simulink model "FullCarLateral"  (R2023b)
settings: Solver=FixedStepAuto  StartTime=0.0  StopTime=30  FixedStep=dt  MaxStep=0.001  RelTol=1e-3
model workspace (MAT data in the model file):
  AMU : Simulink.Signal (value not decoded)
  EPSILON : Simulink.Signal (value not decoded)
  FZO : Simulink.Signal (value not decoded)
  LCX : Simulink.Signal (value not decoded)
  LCY : Simulink.Signal (value not decoded)
  LCZ : Simulink.Signal (value not decoded)
  LEX : Simulink.Signal (value not decoded)
  LEY : Simulink.Signal (value not decoded)
  LFZO : Simulink.Signal (value not decoded)
  LHX : Simulink.Signal (value not decoded)
  LHY : Simulink.Signal (value not decoded)
  LKXKAPPA : Simulink.Signal (value not decoded)
  LKYALPHA : Simulink.Signal (value not decoded)
  LKYGAMMA : Simulink.Signal (value not decoded)
  LKZGAMMA : Simulink.Signal (value not decoded)
  LMR : Simulink.Signal (value not decoded)
  LMUV : Simulink.Signal (value not decoded)
  LMUX : Simulink.Signal (value not decoded)
  LMUXAST : Simulink.Signal (value not decoded)
  LMUXPRIME : Simulink.Signal (value not decoded)
  LMUY : Simulink.Signal (value not decoded)
  LMUYAST : Simulink.Signal (value not decoded)
  LMUYPRIME : Simulink.Signal (value not decoded)
  LMX : Simulink.Signal (value not decoded)
  LMY : Simulink.Signal (value not decoded)
  LS : Simulink.Signal (value not decoded)
  LT : Simulink.Signal (value not decoded)
  LVX : Simulink.Signal (value not decoded)
  LVY : Simulink.Signal (value not decoded)
  LVYKAPPA : Simulink.Signal (value not decoded)
  LXALPHA : Simulink.Signal (value not decoded)
  LYKAPPA : Simulink.Signal (value not decoded)
  PCX1 : Simulink.Signal (value not decoded)
  PCY1 : Simulink.Signal (value not decoded)
  PDX1 : Simulink.Signal (value not decoded)
  PDX2 : Simulink.Signal (value not decoded)
  PDX3 : Simulink.Signal (value not decoded)
  PDY1 : Simulink.Signal (value not decoded)
  PDY2 : Simulink.Signal (value not decoded)
  PDY3 : Simulink.Signal (value not decoded)
  PEX1 : Simulink.Signal (value not decoded)
  PEX2 : Simulink.Signal (value not decoded)
  PEX3 : Simulink.Signal (value not decoded)
  PEX4 : Simulink.Signal (value not decoded)
  PEY1 : Simulink.Signal (value not decoded)
  PEY2 : Simulink.Signal (value not decoded)
  PEY3 : Simulink.Signal (value not decoded)
  PEY4 : Simulink.Signal (value not decoded)
  PEY5 : Simulink.Signal (value not decoded)
  PHX1 : Simulink.Signal (value not decoded)
  PHX2 : Simulink.Signal (value not decoded)
  PHY1 : Simulink.Signal (value not decoded)
  PHY2 : Simulink.Signal (value not decoded)
  PKX1 : Simulink.Signal (value not decoded)
  PKX2 : Simulink.Signal (value not decoded)
  PKX3 : Simulink.Signal (value not decoded)
  PKY1 : Simulink.Signal (value not decoded)
  PKY2 : Simulink.Signal (value not decoded)
  PKY3 : Simulink.Signal (value not decoded)
  PKY4 : Simulink.Signal (value not decoded)
  PKY5 : Simulink.Signal (value not decoded)
  PKY6 : Simulink.Signal (value not decoded)
  PKY7 : Simulink.Signal (value not decoded)
  PVX1 : Simulink.Signal (value not decoded)
  PVX2 : Simulink.Signal (value not decoded)
  PVY1 : Simulink.Signal (value not decoded)
  PVY2 : Simulink.Signal (value not decoded)
  PVY3 : Simulink.Signal (value not decoded)
  PVY4 : Simulink.Signal (value not decoded)
  QBZ1 : Simulink.Signal (value not decoded)
  QBZ10 : Simulink.Signal (value not decoded)
  QBZ2 : Simulink.Signal (value not decoded)
  QBZ3 : Simulink.Signal (value not decoded)
  QBZ5 : Simulink.Signal (value not decoded)
  QBZ6 : Simulink.Signal (value not decoded)
  QBZ9 : Simulink.Signal (value not decoded)
  QCZ1 : Simulink.Signal (value not decoded)
  QDZ1 : Simulink.Signal (value not decoded)
  QDZ10 : Simulink.Signal (value not decoded)
  QDZ11 : Simulink.Signal (value not decoded)
  QDZ2 : Simulink.Signal (value not decoded)
  QDZ3 : Simulink.Signal (value not decoded)
  QDZ4 : Simulink.Signal (value not decoded)
  QDZ6 : Simulink.Signal (value not decoded)
  QDZ7 : Simulink.Signal (value not decoded)
  QDZ8 : Simulink.Signal (value not decoded)
  QDZ9 : Simulink.Signal (value not decoded)
  QEZ1 : Simulink.Signal (value not decoded)
  QEZ2 : Simulink.Signal (value not decoded)
  QEZ3 : Simulink.Signal (value not decoded)
  QEZ4 : Simulink.Signal (value not decoded)
  QEZ5 : Simulink.Signal (value not decoded)
  QHZ1 : Simulink.Signal (value not decoded)
  QHZ2 : Simulink.Signal (value not decoded)
  QHZ3 : Simulink.Signal (value not decoded)
  QHZ4 : Simulink.Signal (value not decoded)
  QSX1 : Simulink.Signal (value not decoded)
  QSX2 : Simulink.Signal (value not decoded)
  QSX3 : Simulink.Signal (value not decoded)
  QX1 : Simulink.Signal (value not decoded)
  QX2 : Simulink.Signal (value not decoded)
  QX3 : Simulink.Signal (value not decoded)
  QX4 : Simulink.Signal (value not decoded)
  QX5 : Simulink.Signal (value not decoded)
  QX6 : Simulink.Signal (value not decoded)
  RBX1 : Simulink.Signal (value not decoded)
  RBX2 : Simulink.Signal (value not decoded)
  RBX3 : Simulink.Signal (value not decoded)
  RBY1 : Simulink.Signal (value not decoded)
  RBY2 : Simulink.Signal (value not decoded)
  RBY3 : Simulink.Signal (value not decoded)
  RBY4 : Simulink.Signal (value not decoded)
  RCX1 : Simulink.Signal (value not decoded)
  RCY1 : Simulink.Signal (value not decoded)
  REX1 : Simulink.Signal (value not decoded)
  REX2 : Simulink.Signal (value not decoded)
  REY1 : Simulink.Signal (value not decoded)
  REY2 : Simulink.Signal (value not decoded)
  RHX1 : Simulink.Signal (value not decoded)
  RHY1 : Simulink.Signal (value not decoded)
  RHY2 : Simulink.Signal (value not decoded)
  RO : Simulink.Signal (value not decoded)
  RVY1 : Simulink.Signal (value not decoded)
  RVY2 : Simulink.Signal (value not decoded)
  RVY3 : Simulink.Signal (value not decoded)
  RVY4 : Simulink.Signal (value not decoded)
  RVY5 : Simulink.Signal (value not decoded)
  RVY6 : Simulink.Signal (value not decoded)
  SSZ1 : Simulink.Signal (value not decoded)
  SSZ2 : Simulink.Signal (value not decoded)
  SSZ3 : Simulink.Signal (value not decoded)
  SSZ4 : Simulink.Signal (value not decoded)
  VCX : Simulink.Signal (value not decoded)
  ZETA0 : Simulink.Signal (value not decoded)
  ZETA1 : Simulink.Signal (value not decoded)
  ZETA2 : Simulink.Signal (value not decoded)
  ZETA3 : Simulink.Signal (value not decoded)
  ZETA4 : Simulink.Signal (value not decoded)
  ZETA5 : Simulink.Signal (value not decoded)
  ZETA6 : Simulink.Signal (value not decoded)
  ZETA7 : Simulink.Signal (value not decoded)
  ZETA8 : Simulink.Signal (value not decoded)
values from neighbouring files (symbols this model uses):
  A = load('PSS LATERAL FORCE COEFFS.mat').A    [FullCarLateralParams.m]
  B = load('PSS ALIGNING TORQUE COEFFS.mat').B    [FullCarLateralParams.m]
  b = 0.085    [FullCarLateralParams.m]
  C = load('COMBINED OVERTURNING MOMENT COEFFS.mat').C    [FullCarLateralParams.m]
  c_roll = 0.1    [FullCarLateralParams.m]
  cD = 1.23    [FullCarLateralParams.m]
  cL = 3.71    [FullCarLateralParams.m]
  D = load('PLS LONGITUDINAL FORCE COEFFS.mat').D    [FullCarLateralParams.m]
  dt = 0.001    [FullCarLateralParams.m]
  E = load('COMBINED LONGITUDINAL FORCE COEFFS.mat').E    [FullCarLateralParams.m]
  e_FL = atan(tf/lf)    [FullCarLateralParams.m]
  e_FR = atan(lf/tf)    [FullCarLateralParams.m]
  e_RL = atan(lr/tr)    [FullCarLateralParams.m]
  e_RR = atan(tr/lr)    [FullCarLateralParams.m]
  F = load('COMBINED LATERAL FORCE COEFFS.mat').F    [FullCarLateralParams.m]
  frontalA = 1    [FullCarLateralParams.m]
  g = 9.81    [FullCarLateralParams.m]
  G = load('COMBINED ALIGNING TORQUE COEFFS.mat').G    [FullCarLateralParams.m]
  gearboxEff = 0.95    [FullCarLateralParams.m]
  GR = 11.86    [FullCarLateralParams.m]
  hCG = 0.2    [FullCarLateralParams.m]
  Ix_wheel = (0.07829 + Ix_motor*GR*GR) * Ix_wheel_factor    (= 0.1168307304)    [FullCarLateralParams.m]
  Iz_vehicle = 125    [FullCarLateralParams.m]
  lf = wb - lr    (= 0.755)    [FullCarLateralParams.m]
  lowpassT = 0.05    [FullCarLateralParams.m]
  lr = 0.78    [FullCarLateralParams.m]
  m = 250    [FullCarLateralParams.m]
  motorOmegaLimit = 2094    [FullCarLateralParams.m]
  R_FL = sqrt(tf^2 + lf^2)    [FullCarLateralParams.m]
  R_FR = R_FL    [FullCarLateralParams.m]
  R_RL = sqrt(tr^2 + lr^2)    [FullCarLateralParams.m]
  R_RR = R_RL    [FullCarLateralParams.m]
  R_wheel = 0.2    [FullCarLateralParams.m]
  rho = 1.293    [FullCarLateralParams.m]
  tireFactor_X_Accel = 0.6    [FullCarLateralParams.m]
  tireFactor_X_Brake = 0.6    [FullCarLateralParams.m]
  tireFactor_Y = 1    [FullCarLateralParams.m]
  TLLTD = 0.5    [FullCarLateralParams.m]
  tr = trackWidth / 2    (= 0.6)    [FullCarLateralParams.m]
  trackWidth = 1.2    [FullCarLateralParams.m]
  wb = 1.535    [FullCarLateralParams.m]
  wheelSideBrakeFactor = 1    [FullCarLateralParams.m]
undefined symbols (not defined in the file or in its folder): trackReference
libraries: simulink_extras x11, eeGeneralControl x3, slpidlib x2, simulink x2
(part 6 of 6)

== matlab function FullCarLateral/Car/Tire Model Pacejka 5.2/Pacejka 5.2 FL3 ==
  settings: updateMethod=DISCRETE  sampleTime=dt
  data: SL input; FX output; SA input; FZ input; IA input; FY output; FZO data_store_memory; RO data_store_memory; VCX data_store_memory; PCY1 data_store_memory; PDY1 data_store_memory; PDY2 data_store_memory; PDY3 data_store_memory; PEY1 data_store_memory; PEY2 data_store_memory; PEY3 data_store_memory; PEY4 data_store_memory; PEY5 data_store_memory; PKY1 data_store_memory; PKY2 data_store_memory; PKY3 data_store_memory; PKY4 data_store_memory; PKY5 data_store_memory; PKY6 data_store_memory; PKY7 data_store_memory; PHY1 data_store_memory; PHY2 data_store_memory; PVY1 data_store_memory; PVY2 data_store_memory; PVY3 data_store_memory; PVY4 data_store_memory; PCX1 data_store_memory; PDX1 data_store_memory; PDX2 data_store_memory; PDX3 data_store_memory; PEX1 data_store_memory; PEX2 data_store_memory; PEX3 data_store_memory; PEX4 data_store_memory; PKX1 data_store_memory; PKX2 data_store_memory; PKX3 data_store_memory; PHX1 data_store_memory; PHX2 data_store_memory; PVX1 data_store_memory; PVX2 data_store_memory; QBZ1 data_store_memory; QBZ2 data_store_memory; QBZ3 data_store_memory; QBZ5 data_store_memory; QBZ6 data_store_memory; QBZ9 data_store_memory; QBZ10 data_store_memory; QCZ1 data_store_memory; QDZ1 data_store_memory; QDZ2 data_store_memory; QDZ3 data_store_memory; QDZ4 data_store_memory; QDZ6 data_store_memory; QDZ7 data_store_memory; QDZ8 data_store_memory; QDZ9 data_store_memory; QDZ10 data_store_memory; QDZ11 data_store_memory; QEZ1 data_store_memory; QEZ2 data_store_memory; QEZ3 data_store_memory; QEZ4 data_store_memory; QEZ5 data_store_memory; QHZ1 data_store_memory; QHZ2 data_store_memory; QHZ3 data_store_memory; QHZ4 data_store_memory; QSX1 data_store_memory; QSX2 data_store_memory; QSX3 data_store_memory; QX1 data_store_memory; QX2 data_store_memory; QX3 data_store_memory; QX4 data_store_memory; QX5 data_store_memory; QX6 data_store_memory; RBX1 data_store_memory; RBX2 data_store_memory; RBX3 data_store_memory; RCX1 data_store_memory; REX1 data_store_memory; REX2 data_store_memory; RHX1 data_store_memory; RBY1 data_store_memory; RBY2 data_store_memory; RBY3 data_store_memory; RBY4 data_store_memory; RCY1 data_store_memory; REY1 data_store_memory; REY2 data_store_memory; RHY1 data_store_memory; RHY2 data_store_memory; RVY1 data_store_memory; RVY2 data_store_memory; RVY3 data_store_memory; RVY4 data_store_memory; RVY5 data_store_memory; RVY6 data_store_memory; SSZ1 data_store_memory; SSZ2 data_store_memory; SSZ3 data_store_memory; SSZ4 data_store_memory; ZETA0 data_store_memory; ZETA1 data_store_memory; ZETA2 data_store_memory; ZETA3 data_store_memory; ZETA4 data_store_memory; ZETA5 data_store_memory; ZETA6 data_store_memory; ZETA7 data_store_memory; ZETA8 data_store_memory; EPSILON data_store_memory; LFZO data_store_memory; LCX data_store_memory; LCY data_store_memory; LEX data_store_memory; LEY data_store_memory; LHX data_store_memory; LHY data_store_memory; LVX data_store_memory; LVY data_store_memory; LKYGAMMA data_store_memory; LKZGAMMA data_store_memory; LT data_store_memory; LMR data_store_memory; AMU data_store_memory; LMUX data_store_memory; LMUY data_store_memory; LMUV data_store_memory; LKXKAPPA data_store_memory; LKYALPHA data_store_memory; LMUXAST data_store_memory; LMUYAST data_store_memory; LMUYPRIME data_store_memory; LMUXPRIME data_store_memory; LXALPHA data_store_memory; LYKAPPA data_store_memory; LVYKAPPA data_store_memory; LS data_store_memory; LCZ data_store_memory; LMX data_store_memory; LMY data_store_memory; A input; B input; C input; D input; E input; F input; G input; MZ output
function [FX, FY, MZ] = fcn(SL, SA, FZ, IA, A, B, C, D, E, F, G)

    if (abs(SA) > 20)
        SA = 20 * sign(SA);
    end

    %% INITIALIZE PACEJKA 5.2 VARIABLES, PARAMETERS, AND SCALING FACTORS
    
    % CONVENTION: 
    % SAE FOR TTC TIRE AXIS SYSTEM 
    % ADAPTED SAE FOR PACEJKA MODEL
    
    % !!!!! SEE TTC TIRE AXIS SYSTEM.png FOR SA DIRECTION !!!!!
    % !!!!! SEE PACEJKA AXIS SYSTEM PT1 & 2.png FOR SA DIRECTION !!!!!!
    
    % ALPHA = SA, GAMMA = IA, KAPPA = LONGITUDINAL SLIP
    
    % ALL ANGLES USED IN MODEL PARAM. DETERMINATION = RADIAN
    
    % Variables
    global FZO RO VCX
    
    % PURE SIDE SLIP FY PARAMETERS
    global PCY1 ...
           PDY1 PDY2 PDY3 ...
           PEY1 PEY2 PEY3 PEY4 PEY5...
           PKY1 PKY2 PKY3 PKY4 PKY5 PKY6 PKY7...
           PHY1 PHY2 ...
           PVY1 PVY2 PVY3 PVY4
    
    % PURE LONG. SLIP FX PARAMETERS
    global PCX1 ...
           PDX1 PDX2 PDX3 ...
           PEX1 PEX2 PEX3 PEX4 ...
           PKX1 PKX2 PKX3 ...
           PHX1 PHX2 ...
           PVX1 PVX2
    
    % PURE SIDE SLIP MZ PARAMETERS
    global QBZ1 QBZ2 QBZ3 QBZ5 QBZ6 QBZ9 QBZ10...
           QCZ1 ...
           QDZ1 QDZ2 QDZ3 QDZ4 QDZ6 QDZ7 QDZ8 QDZ9 QDZ10 QDZ11 ...
           QEZ1 QEZ2 QEZ3 QEZ4 QEZ5 ...
           QHZ1 QHZ2 QHZ3 QHZ4
    
    % COMBINED FY DEPENDENT MX PARAMETERS 
    global QSX1 QSX2 QSX3
    
    % COMBINED FY DEPENDENT MX PARAMETERS FROM TEXT SECTION 4.3.5
    global QX1 QX2 QX3 QX4 QX5 QX6
    
    % COMBINED FX PARAMETERS
    global RBX1 RBX2 RBX3 ...
           RCX1 ...
           REX1 REX2 ...
           RHX1
    
    % COMBINED FY PARAMETERS
    global RBY1 RBY2 RBY3 RBY4 ...
           RCY1 ...
           REY1 REY2 ...
           RHY1 RHY2 ...
           RVY1 RVY2 RVY3 RVY4 RVY5 RVY6
    
    % COMBINED MZ PARAMETERS
    global SSZ1 SSZ2 SSZ3 SSZ4
            
    
    % Spin factor (ZETA0 -> ZETA8 = UNITY WHEN NEGLECTING TURN SLIP AND CAMBER REMAINS SMALL)
    global ZETA0 ZETA1 ZETA2 ZETA3 ZETA4 ZETA5 ZETA6 ZETA7 ZETA8
    
    % PREVENT SINGULARITY WHEN DENOMINATOR = 0
    global EPSILON
    
    %Scaling factors
    % Pure slip
    global LFZO LMUX LMUY LMUV LKXKAPPA LKYALPHA LCX LCY...
           LEX LEY LHX LHY LVX LVY LKYGAMMA LKZGAMMA ...
           LT LMR AMU LMUXAST LMUYAST LMUYPRIME LMUXPRIME
    
    % Combined
    global LXALPHA LYKAPPA LVYKAPPA LS
    
    % Other
    global LCZ LMX LMY
    

    %% PACEJKA MF 5.2 PARAM SET, ENSURE THESE ARE EXACTLY THE SAME AS FIRST PARAM SET
    
    % ADHERE TO ADAPTED SAE
    FZO = 1100; % N, nominal load, highest tested normal load
    RO = 0.2032; % m, unloaded tire radius
    
    % VCX ONLY USED FOR SIGN
    VCX = 10; % !! CURRENTLY ONLY CONSIDERING POSITIVE LONGITUDINAL VEL., ARBITRARY MAGNITUDE !!
    
    % PURE SLIP SCALING FACTORS
    LFZO        = 1;
    LMUX        = 1;
    LMUY        = 1;
    LKXKAPPA    = 1;
    LKYALPHA    = 1;
    LCX         = 1;
    LCY         = 1;
    LEX         = 1;
    LEY         = 1;
    LHX         = 1;
    LHY         = 1;
    LVX         = 1;
    LVY         = 1;
    LKYGAMMA    = 1;
    LKZGAMMA    = 1;
    LT          = 1;
    LMR         = 1;
    
    % COMBINED - SCALING FACTOR
    LXALPHA     = 1;
    LYKAPPA     = 1;
    LVYKAPPA    = 1;
    LS          = 1;
    
    % OTHER - SCALING FACTOR
    LMX         = 1;
    
    % Allows simplification
    LMUV        = 0;
    
    % Simplification
    AMU = 10; % Suggested value from text
    LMUXAST = LMUX;
    LMUYAST = LMUY;
    LMUYPRIME = AMU .* LMUYAST ./ (1 + (AMU - 1) .* LMUYAST);
    LMUXPRIME = AMU .* LMUXAST ./ (1 + (AMU - 1) .* LMUXAST);
    
    % Spin Factor
    ZETA0 = 1;
    ZETA1 = 1;
    ZETA2 = 1;
    ZETA3 = 1;
    ZETA4 = 1;
    ZETA5 = 1;
    ZETA6 = 1;
    ZETA7 = 1;
    ZETA8 = 1;
    
    % Not expecting any denominator to become 0
    EPSILON = 0;


    %% GET PURE SLIP COEFFS

    % Load PSS LAT. COEFFS.
    
    PCY1 = A(1);
    PDY1 = A(2);
    PDY2 = A(3);
    PDY3 = A(4);
    PEY1 = A(5);
    PEY2 = A(6);
    PEY3 = A(7);
    PEY4 = A(8);
    PEY5 = A(9);
    PKY1 = A(10);
    PKY2 = A(11);
    PKY3 = A(12);
    PKY4 = A(13); 
    PKY5 = A(14); 
    PKY6 = A(15);
    PKY7 = A(16);
    PHY1 = A(17);
    PHY2 = A(18);
    PVY1 = A(19);
    PVY2 = A(20);
    PVY3 = A(21);
    PVY4 = A(22);

    % LOAD PSS MZ COEFFS
    
    QBZ1    = B(1);
    QBZ2    = B(2);
    QBZ3    = B(3);
    QBZ5    = B(4);
    QBZ6    = B(5);
    QBZ9    = B(6);
    QBZ10   = B(7);
    QCZ1    = B(8);
    QDZ1    = B(9);
    QDZ2    = B(10);
    QDZ3    = B(11);
    QDZ4    = B(12);
    QDZ6    = B(13);
    QDZ7    = B(14);
    QDZ8    = B(15);
    QDZ9    = B(16);
    QDZ10   = B(17);
    QDZ11   = B(18);
    QEZ1    = B(19);
    QEZ2    = B(20);
    QEZ3    = B(21);
    QEZ4    = B(22);
    QEZ5    = B(23);  
    QHZ1    = B(24);
    QHZ2    = B(25);
    QHZ3    = B(26);
    QHZ4    = B(27);


    % LOAD PLS LONG. COEFFS
    
    PCX1 = D(1);
    PDX1 = D(2);
    PDX2 = D(3);
    PDX3 = D(4);
    PEX1 = D(5);
    PEX2 = D(6);
    PEX3 = D(7);
    PEX4 = D(8);
    PKX1 = D(9);
    PKX2 = D(10);
    PKX3 = D(11);
    PHX1 = D(12);
    PHX2 = D(13);
    PVX1 = D(14);
    PVX2 = D(15);


    %% GET COMBINED SLIP COEFFS

    % LOAD COMBINED FX COEFFS.
    
    RBX1 = E(1);
    RBX2 = E(2);
    RBX3 = E(3);
    RCX1 = E(4);
    REX1 = E(5);
    REX2 = E(6);
    RHX1 = E(7);


    % LOAD COMBINED FY COEFFS.
    
    RBY1 = F(1);
    RBY2 = F(2);
    RBY3 = F(3);
    RBY4 = F(4);
    RCY1 = F(5);
    REY1 = F(6);
    REY2 = F(7);
    RHY1 = F(8);
    RHY2 = F(9);
    RVY1 = F(10);
    RVY2 = F(11);
    RVY3 = F(12);
    RVY4 = F(13);
    RVY5 = F(14);
    RVY6 = F(15);


    % LOAD COMBINED MZ COEFFS.
    
    SSZ1 = G(1);
    SSZ2 = G(2);
    SSZ3 = G(3);
    SSZ4 = G(4);

    
    QSX1 = C(1);
    QSX2 = C(2);
    QSX3 = C(3);


    %% GET FORCES

    % RUN FUNCTIONS

    if isnan(SA)
        SA = 0;
    end

    INPUT = [SL, SA, -FZ, IA];

    COMBINED_FY = Pacejka52_COMBINED_FY(F, INPUT);
    COMBINED_FX = Pacejka52_COMBINED_FX(E, INPUT);
    COMBINED_MZ = Pacejka52_COMBINED_MZ(G, INPUT);
    COMBINED_MX = Pacejka52_COMBINED_MX(C, INPUT);

    %% EXTRAPOLATION SCALING
    % KAPPA_EXP_INDS = abs(SL) >= 0.2;
    % 
    % FX_EXTRAP_COEFFS = FX_EXTRAPOLATION_COEFF(SL(KAPPA_EXP_INDS));
    % COMBINED_FX(KAPPA_EXP_INDS) = COMBINED_FX(KAPPA_EXP_INDS) .* FX_EXTRAP_COEFFS;
    % 
    % ALPHA_EXP_INDS = abs(SA) >= 6;
    % FY_EXTRAP_COEFFS = FY_EXTRAPOLATION_COEFF(SA(ALPHA_EXP_INDS));
    % 
    % COMBINED_FY(ALPHA_EXP_INDS) = COMBINED_FY(ALPHA_EXP_INDS) .* FY_EXTRAP_COEFFS;
    %%

    tireForces.COMBINED.FY = COMBINED_FY;
    tireForces.COMBINED.FX = COMBINED_FX;
    tireForces.COMBINED.MZ = COMBINED_MZ;
    tireForces.COMBINED.MX = COMBINED_MX;

    FX = tireForces.COMBINED.FX;
    FY = tireForces.COMBINED.FY;
    MZ = tireForces.COMBINED.MZ;

    if (abs(SA) < 0.25)
        % FY = 0;
        MZ = 0;
    end

== matlab function FullCarLateral/Car/Slip Angle and Corner Velocity/MATLAB Function ==
  data: Vx_B input; Alpha_FL output; Vy_B input; Yaw_Rate input; Delta_Left input; Delta_Right input; Alpha_FR output; Alpha_RL output; Alpha_RR output; LongCornerVel_FL_B output; LongCornerVel_FR_B output; LongCornerVel_RL_B output; LongCornerVel_RR_B output; R_FL input; R_FR input; R_RL input; R_RR input; e_FL input; e_FR input; e_RL input; e_RR input
function [Alpha_FL, Alpha_FR, Alpha_RL, Alpha_RR, LongCornerVel_FL_B, LongCornerVel_FR_B, LongCornerVel_RL_B, LongCornerVel_RR_B] = fcn(Vx_B, Vy_B, Yaw_Rate, Delta_Left, Delta_Right, R_FL, R_FR, R_RL, R_RR, e_FL, e_FR, e_RL, e_RR)

    % CHECK FullCarLateralParams.M FOR SIN AND COS CONVENTION

    %% FL
    num = Vy_B + Yaw_Rate*R_FL*cos(e_FL);
    den = Vx_B + Yaw_Rate*R_FL*sin(e_FL);
    
    test = atan(num/den);
    test1 = atan2(num, den);
    Alpha_FL = -(Delta_Left - test1);
    % Alpha_FL = -(Delta_Left - atan(num/den));
    if (isnan(Alpha_FL))
        if(Delta_Left ~= 0)
            Alpha_FL = -Delta_Left;
        else
            Alpha_FL = 0;
        end
    end
    % Speed_FL = sqrt(num^2 + den^2);
    LongCornerVel_FL_B = den;

    %% FR
    num = Vy_B + Yaw_Rate*R_FR*sin(e_FR);
    den = Vx_B - Yaw_Rate*R_FR*cos(e_FR);
    
    test1 = atan2(num, den);
    Alpha_FR = -(Delta_Right - test1);
    % Alpha_FR = -(Delta_Right - atan(num/den));
    if (isnan(Alpha_FR))
        if(Delta_Right ~= 0)
            Alpha_FR = -Delta_Right;
        else
            Alpha_FR = 0;
        end
    end
    % Speed_FR = sqrt(num^2 + den^2);
    LongCornerVel_FR_B = den;
    
    %% RL
    num = Vy_B - Yaw_Rate*R_RL*sin(e_RL);
    den = Vx_B + Yaw_Rate*R_RL*cos(e_RL);
    
    test1 = atan2(num, den);
    Alpha_RL = test1;
    % Alpha_RL = atan(num/den);
    if (isnan(Alpha_RL))
        Alpha_RL = 0;
    end
    % Speed_RL = sqrt(num^2 + den^2);
    LongCornerVel_RL_B = den;


    %% RR    
    num = Vy_B - Yaw_Rate*R_RR*cos(e_RR);
    den = Vx_B - Yaw_Rate*R_RR*sin(e_RR);

    test1 = atan2(num, den);
    Alpha_RR = test1;
    % Alpha_RR = atan(num/den);
    if (isnan(Alpha_RR))
        Alpha_RR = 0;
    end
    % Speed_RR = sqrt(num^2 + den^2);
    LongCornerVel_RR_B = den;
